simulink model "ActuatorFault"  (R2025b)
settings: Solver=VariableStepAuto  StartTime=0.0  StopTime=30  RelTol=1e-3
values from neighbouring files (symbols this model uses):
  hiddenLayerSize = 2 * inputLayerSize + 1    (= 7)    [Initialization.m]
  inputLayerSize = n + 1    (= 3)    [Initialization.m]
  nnSize = [n, inputLayerSize, hiddenLayerSize, outputLayerSize]    [Initialization.m]
  outputLayerSize = 2    [Initialization.m]
settings Model: Creator=Asus  LastModifiedBy=Asus

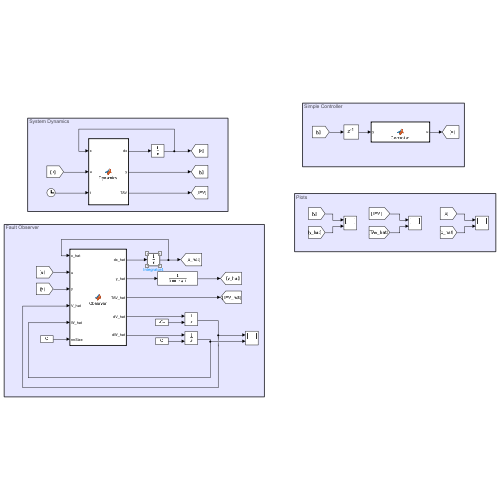
[thumbnail: Simulink's stored preview of the top-level diagram]
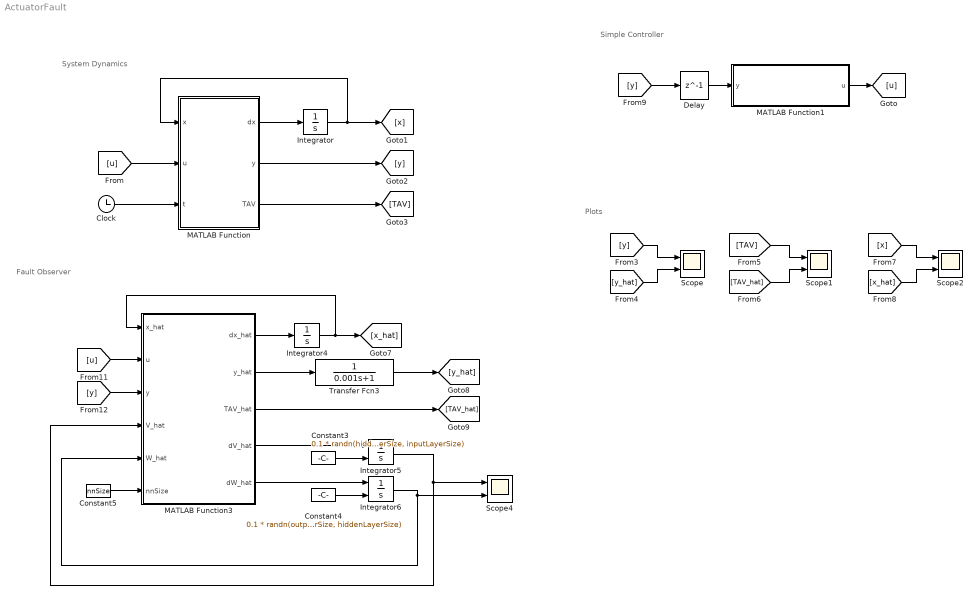
== system ActuatorFault ==
  note: System Dynamics
  note: Simple Controller
  note: Plots
  note: Fault Observer
  Clock : Clock
  Constant3 : Constant  Value=0.1 * randn(hiddenLayerSize, inputLayerSize)
  Constant4 : Constant  Value=0.1 * randn(outputLayerSize, hiddenLayerSize)
  Constant5 : Constant  Value=nnSize
  Delay : Delay  DelayLength=1
  Integrator : Integrator  InitialCondition=[0.5; 0.5]
  Integrator4 : Integrator  InitialCondition=[0.5; 0.5]
  Integrator5 : Integrator  InitialConditionSource=external  InitialCondition=0.1 * randn(hiddenLayerSize, inputLayerSize)
  Integrator6 : Integrator  InitialConditionSource=external  InitialCondition=0.1 * randn(outputLayerSize, hiddenLayerSize)
  MATLAB Function : MATLAB Function  TreatAsAtomicUnit=on
  MATLAB Function1 : MATLAB Function  TreatAsAtomicUnit=on
  MATLAB Function3 : MATLAB Function  TreatAsAtomicUnit=on
  Scope{,1..2,4} (4 alike) : Scope  NumInputPorts=2
      Scope settings: ActiveDisplayYMinimum=-5.1016163714759069  ActiveDisplayYMaximum=5.345014566825129
      Scope1 settings: ActiveDisplayYMinimum=-0.43682015939397312  ActiveDisplayYMaximum=3.38186890659933
      Scope2 settings: ActiveDisplayYMinimum=0.4  ActiveDisplayYMaximum=0.6  DataLoggingVariableName=ScopeData2
      Scope4 settings: ActiveDisplayYMinimum=-1.04838  ActiveDisplayYMaximum=0.78077
  Transfer Fcn3 : TransferFcn  Denominator=[0.001 1]
  wires:
  MATLAB Function1/1(u) -> [u]
  [u] -> MATLAB Function/2(u)
  Clock/1 -> MATLAB Function/3(t)
  Integrator/1 -> MATLAB Function/1(x), [x]
  MATLAB Function/1(dx) -> Integrator/1
  MATLAB Function/2(y) -> [y]
  MATLAB Function/3(TAV) -> [TAV]
  [y] -> Scope/1
  [y_hat] -> Scope/2
  [TAV_hat] -> Scope1/2
  [TAV] -> Scope1/1
  [x_hat] -> Scope2/2
  [x] -> Scope2/1
  Delay/1 -> MATLAB Function1/1(y)
  [y] -> Delay/1
  MATLAB Function3/3(TAV_hat) -> [TAV_hat]
  MATLAB Function3/1(dx_hat) -> Integrator4/1
  Constant3/1 -> Integrator5/2
  [u] -> MATLAB Function3/2(u)
  MATLAB Function3/5(dW_hat) -> Integrator6/1
  MATLAB Function3/4(dV_hat) -> Integrator5/1
  MATLAB Function3/2(y_hat) -> Transfer Fcn3/1
  Constant5/1 -> MATLAB Function3/6(nnSize)
  Integrator6/1 -> Scope4/2, MATLAB Function3/5(W_hat)
  Integrator5/1 -> MATLAB Function3/4(V_hat), Scope4/1
  Integrator4/1 -> MATLAB Function3/1(x_hat), [x_hat]
  [y] -> MATLAB Function3/3(y)
  Transfer Fcn3/1 -> [y_hat]
  Constant4/1 -> Integrator6/2

== matlab function ActuatorFault/MATLAB Function1 ==
  data: u output; y input
function u = Controller(y)
    
    u = - y;

end

== matlab function ActuatorFault/MATLAB Function ==
  data: x input; dx output; y output; u input; t input; TAV output
function [dx, y, TAV] = Dynamics(x, u, t)

    fx  = [x(2); - x(2) - x(1)]; % f(x)
    gx  = [0; 1];                % g(x)
    % TAV = 1 * exp(-0.1*t) * sin(t) * (t > 5);         % actuator fault vector
    TAV = [3; 1];         % actuator fault vector
    % TSV = 0;         % sensor fault vector
    C   = [1, 0];                % output matrix

    dx  = fx + gx * u + TAV;
    y   = C * x;

end

== matlab function ActuatorFault/MATLAB Function3 ==
  data: dx_hat output; x_hat input; u input; y_hat output; y input; V_hat input; W_hat input; TAV_hat output; dV_hat output; dW_hat output; nnSize input
function [dx_hat, y_hat, TAV_hat, dV_hat, dW_hat] = Observer(x_hat, u, y, V_hat, W_hat, nnSize)
        
    fx_hat = [x_hat(2); - x_hat(2) - x_hat(1)]; % f(x_hat)
    gx_hat = [0; 1];                % g(x_hat)
    C      = [1, 0];                % output matrix

    % designing params :
    % Ac    = diag([-1, -1]);
    Ac    = [0, 1; -1, -1];
    eta   = 1 * [70; 70];
    gamma = 1  * [0.1; 0.1];

    % NN kernel function :
    kernel = @(phi) (-1 + 2 ./ (1 + exp(-2 * phi)));

    % NN dimensions :
    n       = nnSize(1); % system order
    nInput  = nnSize(2); % input  layer size
    nHidden = nnSize(3); % hidden layer size
    nOutput = nnSize(4); % output layer size

    % designing observer :
    xNN = [x_hat; u];                       % NN inputs
    TAV_hat = W_hat * kernel(V_hat * xNN); % estimated sensor fault vector 

    % observer output :
    y_hat = C * x_hat;
    y_tilde   = y - y_hat;

    % observer derivative :
    dx_hat = fx_hat + gx_hat * u + TAV_hat;

    % output layer weights adaption law :
    % dW_hat = - eta(1) * (((y_tilde' * C * inv(Ac) * ones(n, 1))' * kernel(V_hat * xNN)))' - ...
    %     gamma(1) * sqrt(y_tilde' * y_tilde) * W_hat'; %#ok
    dW_hat = zeros(size(W_hat));

    % input layer weights adaption law :
    % dV_hat = - eta(2) * y_tilde' * C * inv(Ac) * ones(n, 1) * (W_hat' * (eye(nHidden) - diag((kernel(V_hat * xNN)).^2)))' * tanh(xNN') - ...
    %     gamma(2) * sqrt(y_tilde' * y_tilde) * V_hat; %#ok
    dV_hat = zeros(size(V_hat));

end
